simulink model "W2G_ss_lupa"  (R2021b)
settings: Solver=ode4  StartTime=0  StopTime=10  FixedStep=0.1  MaxStep=0.1  RelTol=1e-3  EnableMultiTasking=on
undefined symbols (not defined in the file): absPower, body, constraint, elecPower, ess, force, fricForce, geometry, gsc, hydroData, Ia, Ib, Ic, mooring, Pgen, Pgrid, pto, ptoSim, Qgrid_lim, simu, Va, Vb, Vc, Vdc, vel, waves, wsc, X, Y, Z
libraries: sm_lib x8, WECSim_Lib_Body_Elements x2, nesl_utility x2, simulink x1, WECSim_Lib_Moorings x1, WECSim_Lib_PTOs x1, WECSim_Lib_Constraints x1
settings Model: Creator=mlawson  LastModifiedBy=alexb
settings SolverCC: ZeroCrossControl=DisableAll  AlgebraicLoopSolver=LineSearch  AutoInsertRateTranBlk=on
settings DataIOCC: SaveFormat=Array  SaveOutput=off  SaveTime=off  ReturnWorkspaceOutputs=off
settings OptimizationCC: LifeSpan=inf  SimCompilerOptimization=on
settings DebuggingCC: UnderspecifiedInitializationDetection=Classic  MergeDetectMultiDrivingBlocksExec=none  SolverPrmCheckMsg=warning  AllowSymbolicDim=off  StateNameClashWarn=warning  SFUnexpectedBacktrackingDiag=warning  SFNoUnconditionalDefaultTransitionDiag=warning  SFMachineParentedDataDiag=warning  ArithmeticOperatorsInVariantConditions=warning
settings HardwareCC: ProdBitPerPointer=32  ProdBitPerSizeT=32  ProdBitPerPtrDiffT=32  ProdLargestAtomicFloat=None  ProdIntDivRoundTo=Undefined  ProdEndianess=Unspecified  ProdWordSize=32  ProdHWDeviceType=32-bit Generic
settings ModelReferenceCC: PropagateSignalLabelsOutOfModel=off
settings SFSimCC: SimUseLocalCustomCode=off  CustomCodeUndefinedFunction=UseInterfaceOnly
settings RTWCC: RTWUseLocalCustomCode=off
settings CodeAppCC: StateflowObjectComments=on
settings GRTTargetCC: TargetLangStandard=C89/C90 (ANSI)
settings ConfigComp: CovMetricSettings=dw  CovSaveCumulativeToWorkspaceVar=on  CovSaveSingleToWorkspaceVar=on  CovExternalEMLEnable=off  CovSFcnEnable=off
settings SimscapeCC: SimscapeNormalizeSystem=off
settings ConfigurationSet: Description=SimMechanics 2G
settings ExplorerConfigSet: SimMechanicsOpenEditorOnUpdate=off  InternalSimMechanicsExplorerSettings="<ExplorerConfiguration><canonicalview>default</canonicalview><TilePanel><TileInfo><Tiles Columns=\"1\" Count=\"1\" Rows=\"1\"><Column Left=\"2\" Weight=\"1\"/><Column Left=\"1335\"/><Row Top=\"2\" Weight=\"1\"/><Row Top=\"911\"/><Tile Height=\"1\" Width=\"1\" X=\"0\" Y=\"0\"/></Tiles></TileInfo><SceneInfo><SceneViewer><BGColor><R>0.60000002384185791</R><G>0.60000002384185791</G><B>0.60000002384185791</B></BGColor><Camera><Position><X>365.37645888990272</X><Y>-369.82486814446582</Y><Z>359.64809521743916</Z></Position><Center><X>-6.7351450971904585</X><Y>2.2867358426280204</Y><Z>-12.463508769654169</Z></Center><Up><X>-0.40824829046386307</X><Y>0.40824829046386307</Y><Z>0.81649658092772615</Z></Up><Left>-57.820127362122818</Left><Right>57.820127362122818</Right><Bottom>-38.308817187253304</Bottom><Top>38.308817187253304</Top></Camera></SceneViewer></SceneInfo></TilePanel></ExplorerConfiguration>"

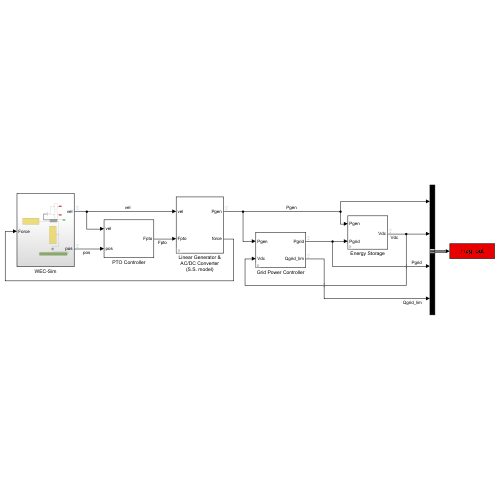
[thumbnail: Simulink's stored preview of the top-level diagram]
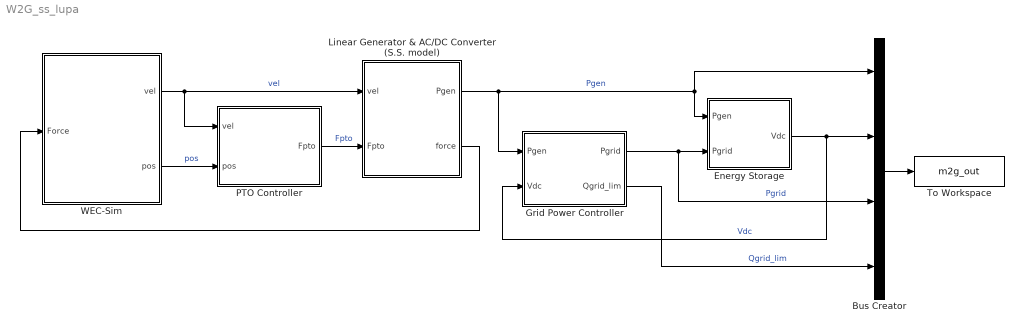
== system W2G_ss_lupa ==
  Bus Creator : BusCreator  Inputs=Pgen,Vdc,Pgrid,Qgrid_lim
  Energy Storage : Subsystem  mask{Vdc_0=ess.Vdc_0, C=ess.C}
      mask prompts: Vdc_0 "Initial Voltage"; C "Capacitance (C):"
      mask DialogControl DescTextVar_copy Prompt: Uses classical SC model.
      mask DialogControl ParamGroupVar Prompt: SC Bank Parameters
  Grid Power Controller : Subsystem  mask{Tavg=gsc.Tavg, Vmag=gsc.Vmag, Ilim=gsc.Ilim, Prated=gsc.Prated, Vdc_nom=ess.Vdc_0, Vdc_del=ess.Vdc_del, kp_v=gsc.kp, ki_v=gsc.ki}
      mask prompts: Tavg "Averaging Time Constant (s):"; Vmag "Grid voltage magnitude (V):"; Ilim "GSC current limit (A):"; Prated "GSC rated power (W):"; Vdc_nom "DC link nominal voltage (V):"; Vdc_del "DC link voltage deviation maximum (V):"; kp_v "Voltage regulator proportional gain:"; ki_v "Voltage regulator integral gain:"
  Linear Generator & AC/DC Converter (S.S. model) : Subsystem  mask{ptoSim=ptoSim.directLinearGenerator(1)}
      mask prompts: ptoSim "Machine Name"
  PTO Controller : Subsystem
  To Workspace : ToWorkspace  VariableName=m2g_out  SaveFormat=Timeseries  SampleTime=-1
  WEC-Sim : Subsystem
  wires:
  WEC-Sim/1(vel) -> PTO Controller/1(vel), Linear Generator & AC/DC Converter (S.S. model)/1(vel)  "vel"
  Linear Generator & AC/DC Converter (S.S. model)/2(force) -> WEC-Sim/1(Force)
  Linear Generator & AC/DC Converter (S.S. model)/1(Pgen) -> Grid Power Controller/1(Pgen), Bus Creator/1, Energy Storage/1(Pgen)  "Pgen"
  Grid Power Controller/1(Pgrid) -> Bus Creator/3, Energy Storage/2(Pgrid)  "Pgrid"
  Grid Power Controller/2(Qgrid_lim) -> Bus Creator/4  "Qgrid_lim"
  Energy Storage/1(Vdc) -> Grid Power Controller/2(Vdc), Bus Creator/2  "Vdc"
  WEC-Sim/2(pos) -> PTO Controller/2(pos)  "pos"
  PTO Controller/1(Fpto) -> Linear Generator & AC/DC Converter (S.S. model)/2(Fpto)  "Fpto"
  Bus Creator/1 -> To Workspace/1

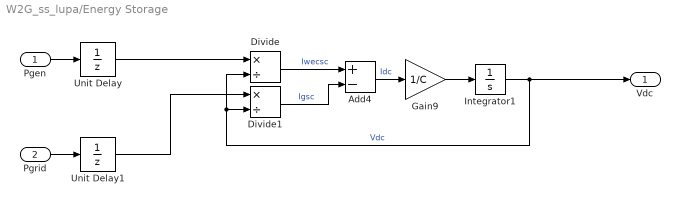
== system W2G_ss_lupa/Energy Storage ==
  Pgen : Inport
  Pgrid : Inport  Port=2
  Add4 : Sum  Inputs=+-
  Divide : Product  Inputs=*/
  Divide1 : Product  Inputs=*/
  Gain9 : Gain  Gain=1/C
  Integrator1 : Integrator  InitialCondition=Vdc_0
  Unit Delay : UnitDelay  SampleTime=-1  HasFrameUpgradeWarning=on
  Unit Delay1 : UnitDelay  SampleTime=-1  HasFrameUpgradeWarning=on
  Vdc : Outport
  wires:
  Pgen/1 -> Unit Delay/1
  Add4/1 -> Gain9/1  "Idc"
  Divide/1 -> Add4/1  "Iwecsc"
  Gain9/1 -> Integrator1/1
  Integrator1/1 -> Vdc/1, Divide1/2, Divide/2  "Vdc"
  Divide1/1 -> Add4/2  "Igsc"
  Pgrid/1 -> Unit Delay1/1
  Unit Delay/1 -> Divide/1
  Unit Delay1/1 -> Divide1/1

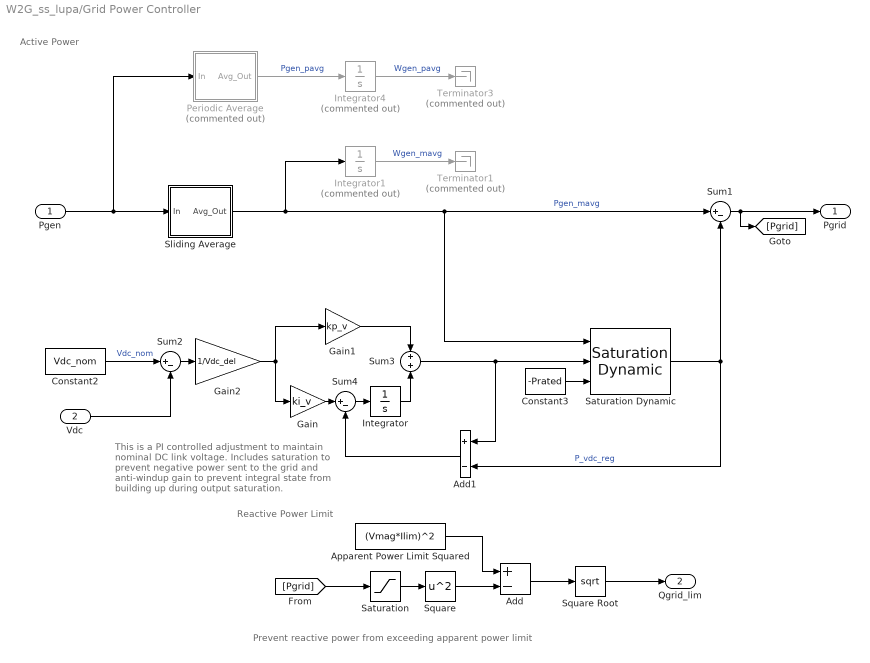
== system W2G_ss_lupa/Grid Power Controller ==
  note: This is a PI controlled adjustment to maintain nominal DC link voltage. Includes saturation to prevent negative power sent to the grid and anti-windup gain to prevent integral state from building up during output saturation.
  note: Reactive Power Limit
  note: Active Power
  note: Prevent reactive power from exceeding apparent power limit
  Pgen : Inport
  Vdc : Inport  Port=2
  Add : Sum  Inputs=+-
  Add1 : Sum  Inputs=+-
  Apparent Power Limit Squared : Constant  Value=(Vmag*Ilim)^2
  Constant2 : Constant  Value=Vdc_nom
  Constant3 : Constant  Value=-Prated
  Gain : Gain  Gain=ki_v
  Gain1 : Gain  Gain=kp_v
  Gain2 : Gain  Gain=1/Vdc_del
  Integrator : Integrator
  Integrator1 : Integrator  Commented=on
  Integrator4 : Integrator  Commented=on
  Periodic Average : Subsystem  Commented=on  mask{Tsample=Tavg}
      mask prompts: Tsample "Sampling Period (s):"
  Saturation : Saturate  UpperLimit=Vmag*Ilim  LowerLimit=-Vmag*Ilim
  Saturation Dynamic : simulink/Discontinuities/Saturation Dynamic  OutMin=[]  OutMax=[]  OutDataTypeStr=Inherit: Same as second input  OutDataType=fixdt(1, 16)  OutScaling=2^-10  DoSatur=off
  Sliding Average : Subsystem  mask{Tsample=Tavg, dt=simu.dt}
      mask prompts: Tsample "Sampling Period (s):"; dt "Simulation Time Step (s):"
  Square : Math  Operator=square  SaturateOnIntegerOverflow=on
  Square Root : Sqrt  SaturateOnIntegerOverflow=on
  Sum1 : Sum  Inputs=|+-
  Sum2 : Sum  Inputs=|+-
  Sum3 : Sum
  Sum4 : Sum  Inputs=|+-
  Terminator1 : Terminator  Commented=on
  Terminator3 : Terminator  Commented=on
  Pgrid : Outport
  Qgrid_lim : Outport  Port=2
  wires:
  Pgen/1 -> Periodic Average/1(In), Sliding Average/1(In)
  Integrator4/1 -> Terminator3/1  "Wgen_pavg"
  Integrator1/1 -> Terminator1/1  "Wgen_mavg"
  Sliding Average/1(Avg_Out) -> Saturation Dynamic/1, Sum1/1, Integrator1/1  "Pgen_mavg"
  Periodic Average/1(Avg_Out) -> Integrator4/1  "Pgen_pavg"
  Add/1 -> Square Root/1
  Square/1 -> Add/2
  Saturation/1 -> Square/1
  Square Root/1 -> Qgrid_lim/1
  Apparent Power Limit Squared/1 -> Add/1
  Sum1/1 -> [Pgrid], Pgrid/1
  [Pgrid] -> Saturation/1
  Constant2/1 -> Sum2/1  "Vdc_nom"
  Constant3/1 -> Saturation Dynamic/3
  Sum3/1 -> Add1/1, Saturation Dynamic/2
  Gain1/1 -> Sum3/1
  Integrator/1 -> Sum3/2
  Saturation Dynamic/1 -> Add1/2, Sum1/2  "P_vdc_reg"
  Vdc/1 -> Sum2/2
  Sum2/1 -> Gain2/1
  Gain2/1 -> Gain1/1, Gain/1
  Gain/1 -> Sum4/1
  Sum4/1 -> Integrator/1
  Add1/1 -> Sum4/2

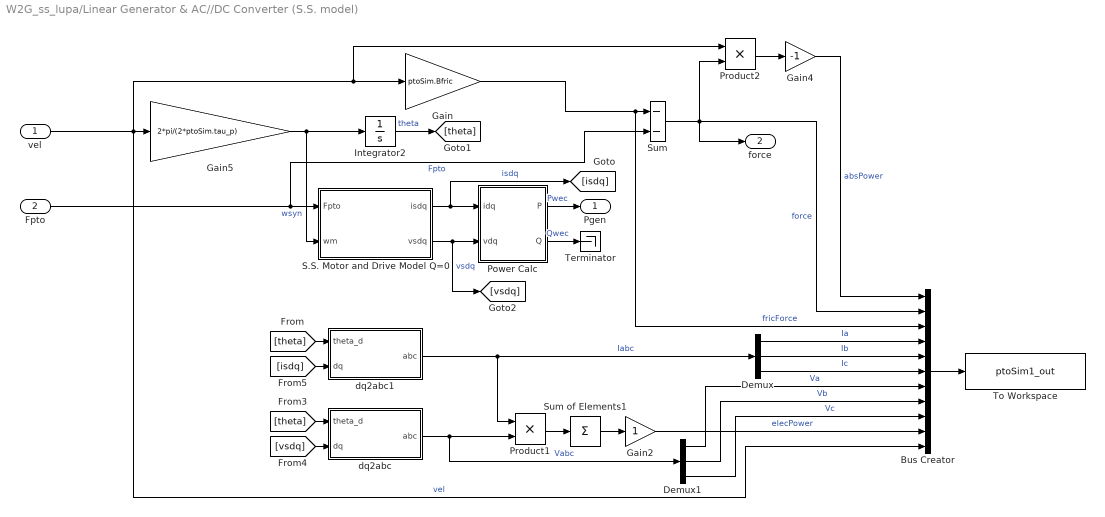
== system W2G_ss_lupa/Linear Generator & AC//DC Converter (S.S. model) ==
  vel : Inport
  Fpto : Inport  Port=2
  Bus Creator : BusCreator  Inputs=absPower,force,fricForce,Ia,Ib,Ic,Va,Vb,Vc,elecPower,vel
  Demux : Demux  Outputs=3
  Demux1 : Demux  Outputs=3
  Gain : Gain  Gain=ptoSim.Bfric
  Gain2 : Gain
  Gain4 : Gain  Gain=-1
  Gain5 : Gain  Gain=2*pi/(2*ptoSim.tau_p)
  Integrator2 : Integrator  InitialCondition=ptoSim.theta_d_0
  Power Calc : Subsystem
  Product1 : Product
  Product2 : Product
  S.S. Motor and Drive Model Q=0 : Subsystem
  Sum : Sum  Inputs=--
  Sum of Elements1 : Sum  Inputs=+
  Terminator : Terminator
  To Workspace : ToWorkspace  VariableName=ptoSim1_out  SaveFormat=Structure With Time  SampleTime=simu.dtOut
  dq2abc : Subsystem
  dq2abc1 : Subsystem
  Pgen : Outport
  force : Outport  Port=2
  wires:
  Gain/1 -> Sum/1, Bus Creator/3  "fricForce"
  S.S. Motor and Drive Model Q=0/2(vsdq) -> [vsdq], Power Calc/2(vdq)  "vsdq"
  Sum/1 -> Product2/2, force/1, Bus Creator/2  "force"
  Sum of Elements1/1 -> Gain2/1
  Integrator2/1 -> [theta]  "theta"
  vel/1 -> Gain/1, Product2/1, Bus Creator/11, Gain5/1  "vel"
  Gain2/1 -> Bus Creator/10  "elecPower"
  Product1/1 -> Sum of Elements1/1
  dq2abc/1(abc) -> Demux1/1, Product1/2  "Vabc"
  Demux1/3 -> Bus Creator/9  "Vc"
  Demux1/2 -> Bus Creator/8  "Vb"
  Demux/3 -> Bus Creator/6  "Ic"
  Gain5/1 -> Integrator2/1, S.S. Motor and Drive Model Q=0/2(wm)  "wsyn"
  Demux1/1 -> Bus Creator/7  "Va"
  Demux/1 -> Bus Creator/4  "Ia"
  S.S. Motor and Drive Model Q=0/1(isdq) -> Power Calc/1(idq), [isdq]  "isdq"
  Bus Creator/1 -> To Workspace/1
  Demux/2 -> Bus Creator/5  "Ib"
  dq2abc1/1(abc) -> Product1/1, Demux/1  "Iabc"
  Gain4/1 -> Bus Creator/1  "absPower"
  Product2/1 -> Gain4/1
  Power Calc/2(Q) -> Terminator/1  "Qwec"
  Power Calc/1(P) -> Pgen/1  "Pwec"
  [theta] -> dq2abc1/1(theta_d)
  [theta] -> dq2abc/1(theta_d)
  [vsdq] -> dq2abc/2(dq)
  [isdq] -> dq2abc1/2(dq)
  Fpto/1 -> S.S. Motor and Drive Model Q=0/1(Fpto), Sum/2  "Fpto"

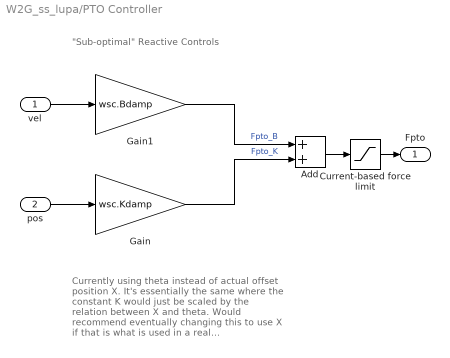
== system W2G_ss_lupa/PTO Controller ==
  note: "Sub-optimal" Reactive Controls
  note: Currently using theta instead of actual offset position X. It's essentially the same where the constant K would just be scaled by the relation between X and theta. Would recommend eventually changing this to use X if that is what is used in a real implementation.
  vel : Inport
  pos : Inport  Port=2
  Add : Sum
  Current-based force limit : Saturate  UpperLimit=wsc.Fpto_lim  LowerLimit=-wsc.Fpto_lim
  Gain : Gain  Gain=wsc.Kdamp
  Gain1 : Gain  Gain=wsc.Bdamp
  Fpto : Outport
  wires:
  Gain1/1 -> Add/1  "Fpto_B"
  Gain/1 -> Add/2  "Fpto_K"
  vel/1 -> Gain1/1
  pos/1 -> Gain/1
  Add/1 -> Current-based force limit/1
  Current-based force limit/1 -> Fpto/1

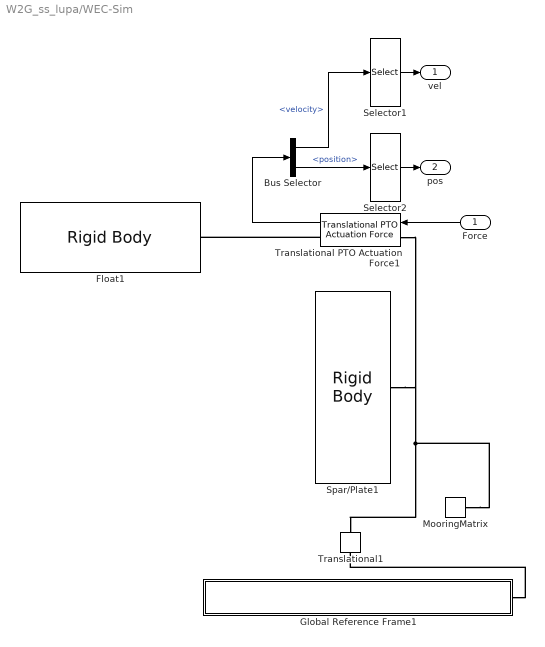
== system W2G_ss_lupa/WEC-Sim ==
  Force : Inport
  Bus Selector : BusSelector  OutputSignals=velocity,position
  Float1 : WECSim_Lib_Body_Elements/Rigid Body  body=body(1)  h5File=hydroData/*.h5  geometryFile=geometry/*.stl  mass=0  inertia=0 0 0  nonHydro=0  nonlinearHydro=0  centerGravity=0 0 0  centerBuoyancy=0 0 0  dof=6  volume=0  displacement=0 0 0  axis=0 1 0  angle=0  option=0  cd=0 0 0  ca=0 0 0  area=0 0 0  VME=0  rgME=0 0 0  z=0 0 1
      settings: SourceProductName=WEC-Sim
  Global Reference Frame1 : Subsystem  AncestorBlock=WECSim_Lib_Frames/Global Reference Frame  StopFcn=%run('stopWecSim')  mask(Frames){waves=waves, simu=simu, InputMethod=Input File, InputFile=wecSimInputFile.m, mode=normal, explorer=off, solver=ode4, startTime=0, rampTime=100, endTime=400, dt=0.1, cicEndTime=60, stateSpace=0, WaveClass=regular, height=2.5, period=8, elevationFile=NOT DEFINED, spectrumFile=NOT DEFINED, direction=0, spread=1, spectrumType=NOT DEFINED, phaseSeed=0, option=EqualEnergy}
      mask prompts: waves "Wave Class Name"; simu "Simulation Class Name"; InputMethod "Parameter Input Method"; mode "Simulation Mode:"; explorer "SimMechanics Explorer:"; solver "SimSolver:"; startTime "Start Time [s]:"; rampTime "Ramp Time [s]:"; endTime "End Time [s]:"; dt "Step Size [s]:"; cicEndTime "CI Time [s]:"; stateSpace "Turn on State Space"; WaveClass "Select Wave Class:"; height "Wave Height [m]:"; period "Wave Period [s]:"; direction "Wave Direction [deg]:"; spread "Wave Spread [0-1]:"; spectrumType "Wave Spectrum Type:"; phaseSeed "Phase Seed:"; option "Frequency Discretization:"
      mask help:
      | This block contains Global References, including solver configurations, free surface and seabed description, and simulation time.
      | It uses the following fields from the Simulation and Wave classes:
      |
      | Simulation Class:
      |     .endTime
      |     .dt
      |     .domainSize
      |
      | Wave Class:
      |     .waterDepth
      mask Help:
      | This block contains Global References, including solver configurations, free surface and seabed description, and simulation time.
      | It uses the following fields from the Simulation and Wave classes:
      | 
      | Simulation Class:
      |     .endTime
      |     .dt
      |     .domainSize
      | 
      | Wave Class:
      |     .waterDepth
      mask TypeOptions InputMethod: Input File | Custom Parameters
      mask Callback InputMethod: inputOrCustomCallback(gcbh)
      mask TypeOptions mode: normal | accelerator | rapid-accelerator
      mask TypeOptions explorer: on | off
      mask TypeOptions solver: ode4 | ode45
      mask TypeOptions stateSpace: 0 | 1
      mask TypeOptions WaveClass: noWaveCIC | regular | regularCIC | irregular | spectrumImport | etaImport
      mask Callback WaveClass: waveClassCallback(gcbh)
      mask TypeOptions spectrumType: PM | JS | NOT DEFINED
      mask TypeOptions option: EqualEnergy | Traditional
      mask DialogControl InputFileGroup Prompt: Input File
      mask DialogControl InFileButton Prompt: Select File
      mask DialogControl InFileButton Callback: inFileButtonCallback(gcbh)
      mask DialogControl CustomParameterGroup Prompt: Custom Parameters
      mask DialogControl LoadParam Prompt: Load parameters from Input File
      mask DialogControl LoadParam Callback: loadInputFileCallback(gcbh)
      mask DialogControl SimData Prompt: Simulation Data
      mask DialogControl WaveInfo Prompt: Wave Information
      mask DialogControl ETAbutton Prompt: Select etaData.mat file
      mask DialogControl ETAbutton Callback: etaButtonCallback(gcbh)
      mask DialogControl SpecButton Prompt: Select spectrumData.mat file
      mask DialogControl SpecButton Callback: spectrumButtonCallback(gcbh)
      mask Display: fprintf('Active Method: \n%s',get_param(gcbh,'InputMethod'))
  MooringMatrix : WECSim_Lib_Moorings/MooringMatrix  mooring=mooring(1)  loc=0 0 0  preTension=[0 0 0 0 0 0]  stiffness={ '0', '0', '0', '0', '0', '0'; '0', '0', '0', '0', '0', '0'; '0', '0', '0', '0', '0', '0'; '0', '0', '0', '0', '0', '0'; '0', '0', '0', '0', '0', '0'; '0', '0', '0', '0', '0', '0' }  damping={ '0', '0', '0', '0', '0', '0'; '0', '0', '0', '0', '0', '0'; '0', '0', '0', '0', '0', '0'; '0', '0', '0', '0', '0', '0'; '0', '0', '0', '0', '0', '0'; '0', '0', '0', '0', '0', '0' }
      settings: AttributesFormatString=%<mooring>
  Selector1 : Selector  InputPortWidth=6  IndexOptions=Index vector (dialog)  Indices=3  OutputSizes=1
  Selector2 : Selector  InputPortWidth=6  IndexOptions=Index vector (dialog)  Indices=3  OutputSizes=1
  Spar/Plate1 : WECSim_Lib_Body_Elements/Rigid Body  body=body(2)  h5File=hydroData/*.h5  geometryFile=geometry/*.stl  mass=0  inertia=0 0 0  nonHydro=0  nonlinearHydro=0  centerGravity=0 0 0  centerBuoyancy=0 0 0  dof=6  volume=0  displacement=0 0 0  axis=0 1 0  angle=0  option=0  cd=0 0 0  ca=0 0 0  area=0 0 0  VME=0  rgME=0 0 0  z=0 0 1
      settings: SourceProductName=WEC-Sim
  Translational PTO Actuation Force1 : WECSim_Lib_PTOs/Translational PTO Actuation Force  pto=pto(1)  loc="0  0  0"  stiffness=0  damping=0  equilibriumPosition=0  pretension=0  displacement=0 0 0  y=0 1 0  z=0 0 1  upperLimitSpecify=off  upperLimitBound=0  upperLimitTransitionRegionWidth=0  upperLimitStiffness=0  upperLimitDamping=0  lowerLimitSpecify=off  lowerLimitBound=0  lowerLimitTransitionRegionWidth=0  lowerLimitStiffness=0  lowerLimitDamping=0
      settings: AttributesFormatString=%<pto>  SourceProductName=WEC-Sim
  Translational1 : WECSim_Lib_Constraints/Translational  constraint=constraint(1)  loc="0  0  0"  displacement=0 0 0  y=0 1 0  z=0 0 1  upperLimitSpecify=off  upperLimitBound=0  upperLimitTransitionRegionWidth=0  upperLimitStiffness=0  upperLimitDamping=0  lowerLimitSpecify=off  lowerLimitBound=0  lowerLimitTransitionRegionWidth=0  lowerLimitStiffness=0  lowerLimitDamping=0
      settings: AttributesFormatString=%<constraint>  SourceProductName=WEC-Sim
  vel : Outport
  pos : Outport  Port=2
  wires:
  Force/1 -> Translational PTO Actuation Force1/1
  Selector1/1 -> vel/1
  Bus Selector/1 -> Selector1/1  "<velocity>"
  Translational PTO Actuation Force1/1 -> Bus Selector/1
  Bus Selector/2 -> Selector2/1  "<position>"
  Selector2/1 -> pos/1
  connections:
  Spar/Plate1/RConn1 -- Translational PTO Actuation Force1/LConn1 -- MooringMatrix/LConn1 -- Translational1/RConn1
  Translational PTO Actuation Force1/RConn1 -- Float1/RConn1
  Global Reference Frame1/RConn1 -- Translational1/LConn1

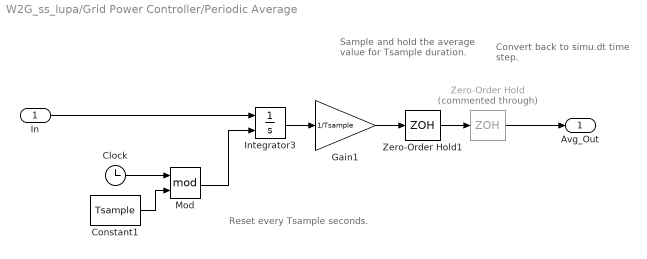
== system W2G_ss_lupa/Grid Power Controller/Periodic Average ==
  note: Reset every Tsample seconds.
  note: Convert back to simu.dt time step.
  note: Sample and hold the average value for Tsample duration.
  In : Inport
  Clock : Clock
  Constant1 : Constant  Value=Tsample
  Gain1 : Gain  Gain=1/Tsample
  Integrator3 : Integrator  ExternalReset=rising
  Mod : Math  Operator=mod  OutputSignalType=real  SaturateOnIntegerOverflow=on
  Zero-Order Hold : ZeroOrderHold  Commented=through  SampleTime=simu.dt
  Zero-Order Hold1 : ZeroOrderHold  SampleTime=Tsample
  Avg_Out : Outport
  wires:
  Zero-Order Hold/1 -> Avg_Out/1
  Mod/1 -> Integrator3/2
  Zero-Order Hold1/1 -> Zero-Order Hold/1
  Clock/1 -> Mod/1
  Gain1/1 -> Zero-Order Hold1/1
  Integrator3/1 -> Gain1/1
  In/1 -> Integrator3/1
  Constant1/1 -> Mod/2

== system W2G_ss_lupa/Grid Power Controller/Sliding Average ==
  In : Inport
  Discrete FIR Filter : DiscreteFir  Coefficients=ones(1,round(Tsample/dt))/round(Tsample/dt)  SampleTime=dt
  Avg_Out : Outport
  wires:
  In/1 -> Discrete FIR Filter/1
  Discrete FIR Filter/1 -> Avg_Out/1

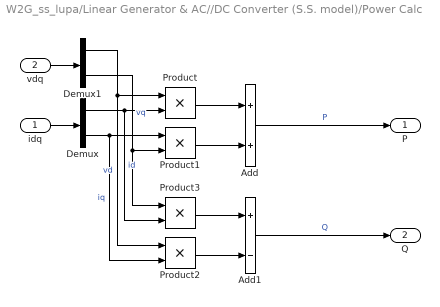
== system W2G_ss_lupa/Linear Generator & AC//DC Converter (S.S. model)/Power Calc ==
  idq : Inport
  vdq : Inport  Port=2
  Add : Sum
  Add1 : Sum  Inputs=+-
  Demux : Demux  Outputs=2
  Demux1 : Demux  Outputs=2
  Product{,1..3} (4 alike) : Product
  P : Outport
  Q : Outport  Port=2
  wires:
  Demux/1 -> Product3/2, Product/2  "id"
  Product1/1 -> Add/2
  Add1/1 -> Q/1  "Q"
  Demux1/2 -> Product1/2, Product3/1  "vq"
  Demux1/1 -> Product/1, Product2/1  "vd"
  Demux/2 -> Product2/2, Product1/1  "iq"
  Product3/1 -> Add1/1
  Product2/1 -> Add1/2
  Product/1 -> Add/1
  Add/1 -> P/1  "P"
  idq/1 -> Demux/1
  vdq/1 -> Demux1/1

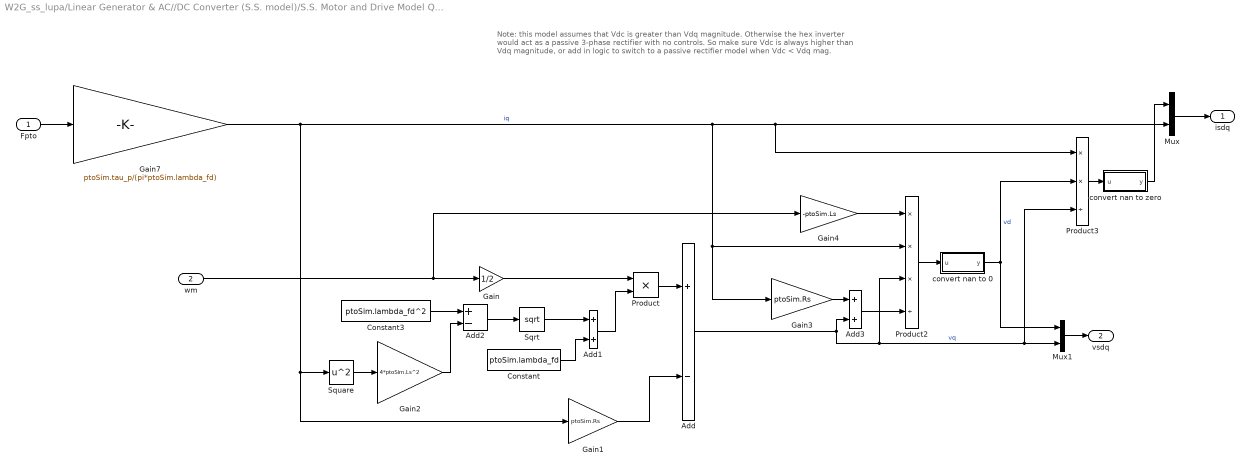
== system W2G_ss_lupa/Linear Generator & AC//DC Converter (S.S. model)/S.S. Motor and Drive Model Q=0 ==
  note: Note: this model assumes that Vdc is greater than Vdq magnitude. Otherwise the hex inverter would act as a passive 3-phase rectifier with no controls. So make sure Vdc is always higher than Vdq magnitude, or add in logic to switch to a passive rectifier model when Vdc < Vdq mag.
  Fpto : Inport
  wm : Inport  Port=2
  Add : Sum  Inputs=+-
  Add1 : Sum
  Add2 : Sum  Inputs=+-
  Add3 : Sum
  Constant : Constant  Value=ptoSim.lambda_fd
  Constant3 : Constant  Value=ptoSim.lambda_fd^2
  Gain : Gain  Gain=1/2
  Gain1 : Gain  Gain=ptoSim.Rs
  Gain2 : Gain  Gain=4*ptoSim.Ls^2
  Gain3 : Gain  Gain=ptoSim.Rs
  Gain4 : Gain  Gain=-ptoSim.Ls
  Gain7 : Gain  Gain=ptoSim.tau_p/(pi*ptoSim.lambda_fd)
  Mux : Mux  Inputs=2
  Mux1 : Mux  Inputs=2
  Product : Product
  Product2 : Product  Inputs=***/
  Product3 : Product  Inputs=**/
  Sqrt : Sqrt  SaturateOnIntegerOverflow=on
  Square : Math  Operator=square  SaturateOnIntegerOverflow=on
  convert nan to 0 : MATLAB Function  TreatAsAtomicUnit=on
  convert nan to zero : MATLAB Function  TreatAsAtomicUnit=on
  isdq : Outport
  vsdq : Outport  Port=2
  wires:
  Fpto/1 -> Gain7/1
  Mux/1 -> isdq/1
  Mux1/1 -> vsdq/1
  Gain7/1 -> Product2/2, Gain3/1, Product3/1, Mux/2, Gain1/1, Square/1  "iq"
  Constant/1 -> Add1/2
  convert nan to 0/1(y) -> Product3/2, Mux1/1  "vd"
  Add/1 -> Product2/3, Product3/3, Mux1/2, Add3/2  "vq"
  convert nan to zero/1(y) -> Mux/1
  Gain1/1 -> Add/2
  Product/1 -> Add/1
  Gain/1 -> Product/1
  Add1/1 -> Product/2
  Sqrt/1 -> Add1/1
  Add2/1 -> Sqrt/1
  Constant3/1 -> Add2/1
  Gain2/1 -> Add2/2
  Product2/1 -> convert nan to 0/1(u)
  Add3/1 -> Product2/4
  Gain3/1 -> Add3/1
  Gain4/1 -> Product2/1
  Product3/1 -> convert nan to zero/1(u)
  Square/1 -> Gain2/1
  wm/1 -> Gain4/1, Gain/1

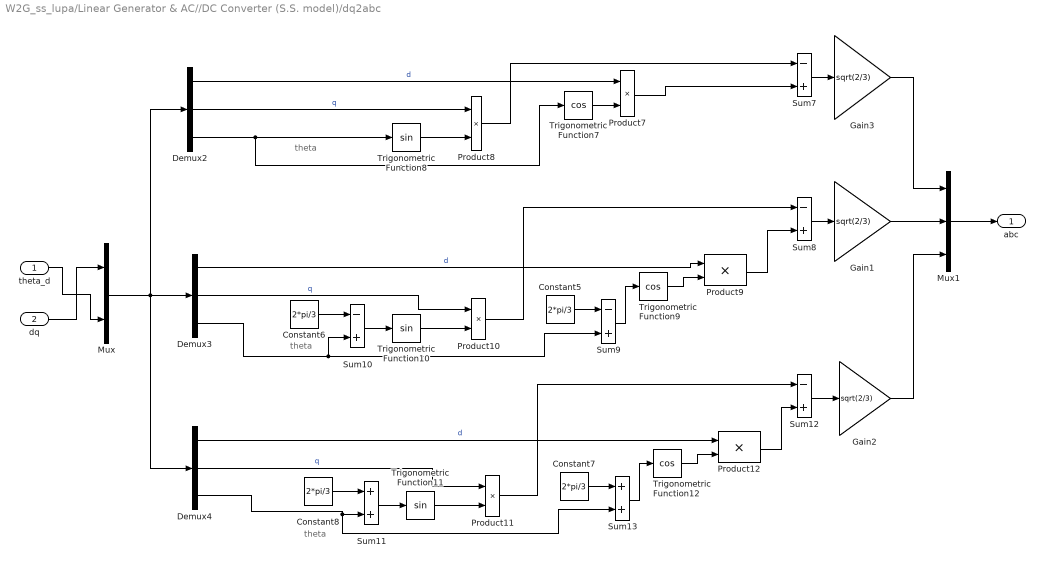
== system W2G_ss_lupa/Linear Generator & AC//DC Converter (S.S. model)/dq2abc ==
  note: theta
  note: theta
  note: theta
  theta_d : Inport
  dq : Inport  Port=2
  Constant{5..8} (4 alike) : Constant  Value=2*pi/3
  Demux2 : Demux  Outputs=3
      settings: DisplayOption=none
  Demux3 : Demux  Outputs=3
      settings: DisplayOption=none
  Demux4 : Demux  Outputs=3
      settings: DisplayOption=none
  Gain1 : Gain  Gain=sqrt(2/3)  SaturateOnIntegerOverflow=on  OutDataTypeStr=Inherit: Same as input  ParamDataTypeStr=Inherit: Same as input
  Gain2 : Gain  Gain=sqrt(2/3)  SaturateOnIntegerOverflow=on  OutDataTypeStr=Inherit: Same as input  ParamDataTypeStr=Inherit: Same as input
  Gain3 : Gain  Gain=sqrt(2/3)  SaturateOnIntegerOverflow=on  OutDataTypeStr=Inherit: Same as input  ParamDataTypeStr=Inherit: Same as input
  Mux : Mux  Inputs=2
  Mux1 : Mux  Inputs=3
  Product{7..12} (6 alike) : Product  InputSameDT=on  SaturateOnIntegerOverflow=on  OutDataTypeStr=Inherit: Same as first input
  Sum{7..10,12} (5 alike) : Sum  Inputs=-+  InputSameDT=on  SaturateOnIntegerOverflow=on  OutDataTypeStr=Inherit: Same as first input
  Sum11 : Sum  InputSameDT=on  SaturateOnIntegerOverflow=on  OutDataTypeStr=Inherit: Same as first input
  Sum13 : Sum  InputSameDT=on  SaturateOnIntegerOverflow=on  OutDataTypeStr=Inherit: Same as first input
  Trigonometric Function10 : Trigonometry
  Trigonometric Function11 : Trigonometry
  Trigonometric Function12 : Trigonometry  Operator=cos
  Trigonometric Function7 : Trigonometry  Operator=cos
  Trigonometric Function8 : Trigonometry
  Trigonometric Function9 : Trigonometry  Operator=cos
  abc : Outport
  wires:
  Constant8/1 -> Sum11/1
  Product7/1 -> Sum7/2
  Gain1/1 -> Mux1/2
  Product9/1 -> Sum8/2
  Sum7/1 -> Gain3/1
  Demux4/2 -> Product11/1  "q"
  Product10/1 -> Sum8/1
  Product11/1 -> Sum12/1
  Sum13/1 -> Trigonometric Function12/1
  Demux2/3 -> Trigonometric Function7/1, Trigonometric Function8/1
  Product12/1 -> Sum12/2
  Constant6/1 -> Sum10/1
  Product8/1 -> Sum7/1
  Mux1/1 -> abc/1
  Demux3/3 -> Sum9/2, Sum10/2
  Demux3/2 -> Product10/1  "q"
  Demux2/2 -> Product8/1  "q"
  dq/1 -> Mux/1
  Trigonometric Function7/1 -> Product7/2
  Constant5/1 -> Sum9/1
  Trigonometric Function12/1 -> Product12/2
  Trigonometric Function10/1 -> Product10/2
  Demux4/1 -> Product12/1  "d"
  Gain2/1 -> Mux1/3
  Demux4/3 -> Sum11/2, Sum13/2
  Demux2/1 -> Product7/1  "d"
  Sum10/1 -> Trigonometric Function10/1
  Gain3/1 -> Mux1/1
  Mux/1 -> Demux3/1, Demux2/1, Demux4/1
  Sum12/1 -> Gain2/1
  theta_d/1 -> Mux/2
  Sum11/1 -> Trigonometric Function11/1
  Trigonometric Function9/1 -> Product9/2
  Sum8/1 -> Gain1/1
  Sum9/1 -> Trigonometric Function9/1
  Demux3/1 -> Product9/1  "d"
  Trigonometric Function8/1 -> Product8/2
  Trigonometric Function11/1 -> Product11/2
  Constant7/1 -> Sum13/1

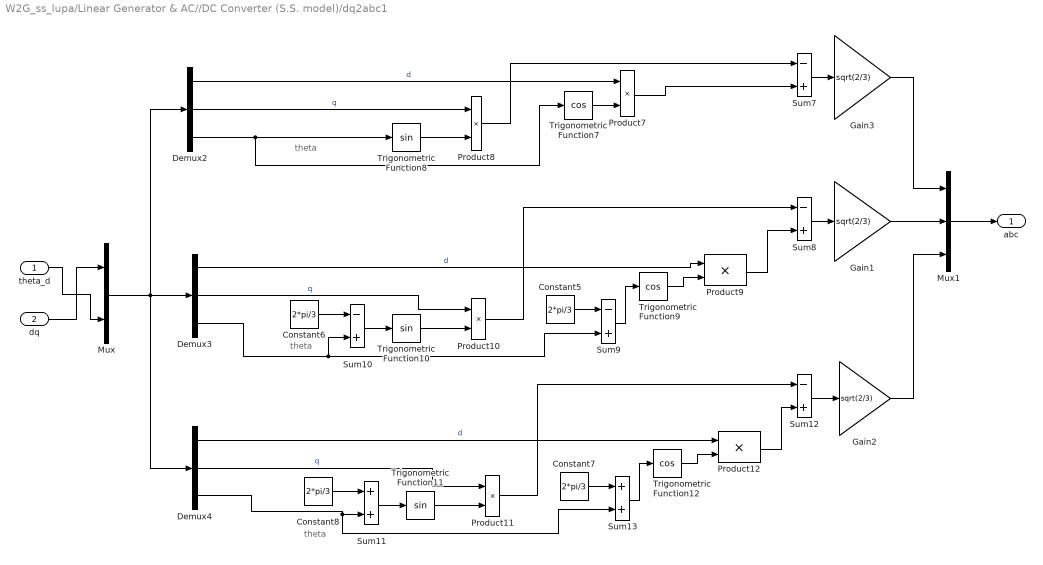
== system W2G_ss_lupa/Linear Generator & AC//DC Converter (S.S. model)/dq2abc1 ==
  note: theta
  note: theta
  note: theta
  theta_d : Inport
  dq : Inport  Port=2
  Constant{5..8} (4 alike) : Constant  Value=2*pi/3
  Demux2 : Demux  Outputs=3
      settings: DisplayOption=none
  Demux3 : Demux  Outputs=3
      settings: DisplayOption=none
  Demux4 : Demux  Outputs=3
      settings: DisplayOption=none
  Gain1 : Gain  Gain=sqrt(2/3)  SaturateOnIntegerOverflow=on  OutDataTypeStr=Inherit: Same as input  ParamDataTypeStr=Inherit: Same as input
  Gain2 : Gain  Gain=sqrt(2/3)  SaturateOnIntegerOverflow=on  OutDataTypeStr=Inherit: Same as input  ParamDataTypeStr=Inherit: Same as input
  Gain3 : Gain  Gain=sqrt(2/3)  SaturateOnIntegerOverflow=on  OutDataTypeStr=Inherit: Same as input  ParamDataTypeStr=Inherit: Same as input
  Mux : Mux  Inputs=2
  Mux1 : Mux  Inputs=3
  Product{7..12} (6 alike) : Product  InputSameDT=on  SaturateOnIntegerOverflow=on  OutDataTypeStr=Inherit: Same as first input
  Sum{7..10,12} (5 alike) : Sum  Inputs=-+  InputSameDT=on  SaturateOnIntegerOverflow=on  OutDataTypeStr=Inherit: Same as first input
  Sum11 : Sum  InputSameDT=on  SaturateOnIntegerOverflow=on  OutDataTypeStr=Inherit: Same as first input
  Sum13 : Sum  InputSameDT=on  SaturateOnIntegerOverflow=on  OutDataTypeStr=Inherit: Same as first input
  Trigonometric Function10 : Trigonometry
  Trigonometric Function11 : Trigonometry
  Trigonometric Function12 : Trigonometry  Operator=cos
  Trigonometric Function7 : Trigonometry  Operator=cos
  Trigonometric Function8 : Trigonometry
  Trigonometric Function9 : Trigonometry  Operator=cos
  abc : Outport
  wires:
  Constant8/1 -> Sum11/1
  Product7/1 -> Sum7/2
  Gain1/1 -> Mux1/2
  Product9/1 -> Sum8/2
  Sum7/1 -> Gain3/1
  Demux4/2 -> Product11/1  "q"
  Product10/1 -> Sum8/1
  Product11/1 -> Sum12/1
  Sum13/1 -> Trigonometric Function12/1
  Demux2/3 -> Trigonometric Function7/1, Trigonometric Function8/1
  Product12/1 -> Sum12/2
  Constant6/1 -> Sum10/1
  Product8/1 -> Sum7/1
  Mux1/1 -> abc/1
  Demux3/3 -> Sum9/2, Sum10/2
  Demux3/2 -> Product10/1  "q"
  Demux2/2 -> Product8/1  "q"
  dq/1 -> Mux/1
  Trigonometric Function7/1 -> Product7/2
  Constant5/1 -> Sum9/1
  Trigonometric Function12/1 -> Product12/2
  Trigonometric Function10/1 -> Product10/2
  Demux4/1 -> Product12/1  "d"
  Gain2/1 -> Mux1/3
  Demux4/3 -> Sum11/2, Sum13/2
  Demux2/1 -> Product7/1  "d"
  Sum10/1 -> Trigonometric Function10/1
  Gain3/1 -> Mux1/1
  Mux/1 -> Demux3/1, Demux2/1, Demux4/1
  Sum12/1 -> Gain2/1
  theta_d/1 -> Mux/2
  Sum11/1 -> Trigonometric Function11/1
  Trigonometric Function9/1 -> Product9/2
  Sum8/1 -> Gain1/1
  Sum9/1 -> Trigonometric Function9/1
  Demux3/1 -> Product9/1  "d"
  Trigonometric Function8/1 -> Product8/2
  Trigonometric Function11/1 -> Product11/2
  Constant7/1 -> Sum13/1

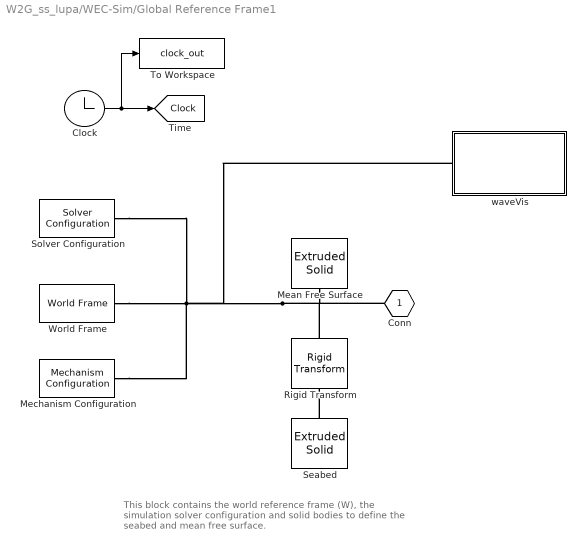
== system W2G_ss_lupa/WEC-Sim/Global Reference Frame1 ==
  note: This block contains the world reference frame (W), the simulation solver configuration and
      | solid bodies to define the seabed and mean free surface.
  Clock : Clock
  Mean Free Surface : sm_lib/Body Elements/Extruded Solid  GraphicAmbientColor=[0.15 0.15 0.15 1.0]  BasedOnType=Density  CenterOfMass=[0 0 0]  CenterOfMassUnits=m  GraphicDiffuseColor=[0.0 0.6 0.8]  ExportConvexHullGeometry=off  ExtrusionCrossSection=[simu.domainSize simu.domainSize; -simu.domainSize simu.domainSize; -simu.domainSize -simu.domainSize; simu.domainSize -simu.domainSize]  ExtrusionCrossSectionUnits=m  Density=1000  DensityUnits=kg/(m^3)  DoExposeReferenceFrame=on  GraphicEmissiveColor=[0.0 0.0 0.0 1.0]  ExportEntireGeometry=off  ExtrusionLength=simu.domainSize/200  ExtrusionLengthUnits=m  ExtrusionType=General  SerializedFrames=<Frames/>  MarkerShape=Sphere  MarkerSize=10  GraphicType=FromGeometry  InertiaType=Custom  Mass=10^20  MassUnits=kg  MomentsOfInertia=[10^20 10^20 10^20]  MomentsOfInertiaUnits=kg*m^2  PolygonNumSides=3  GraphicOpacity=0.3  PolygonOuterRadius=1  PolygonOuterRadiusUnits=m  ProductsOfInertia=[0 0 0]  ProductsOfInertiaUnits=kg*m^2  GraphicShininess=75  GraphicSpecularColor=[0.5 0.5 0.5 1.0]  GraphicVisPropType=SimpleVisualProperties
  Mechanism Configuration : sm_lib/Utilities/Mechanism Configuration  UniformGravity=Constant  GravityVector=[0 0 0]  GravityUnits=m/s^2  LinearizationDelta=0.001  JointModeTransitionNonlinearIterations=2
  Rigid Transform : sm_lib/Frames and Transforms/Rigid Transform  TranslationMethod=Cartesian  TranslationStandardOffset=0  TranslationLengthUnit=m  TranslationStandardAxis=+Z  TranslationCartesianOffset=[0 0 -waves.waterDepth]  TranslationROffset=0  TranslationROffsetUnits=m  TranslationZOffset=0  TranslationZOffsetUnits=m  TranslationThetaOffset=0  TranslationThetaOffsetUnits=deg  RotationMethod=None  RotationAngleUnits=deg  RotationStandardAxis=+Z  RotationAngle=0  RotationArbitraryAxis=[0 0 1]  FollAlignAxisA=+X  BaseAlignAxisA=+Y  FollAlignAxisB=+Y  BaseAlignAxisB=+Z  RotationSequenceAxes=FollowerAxes  RotationSequence=XYX  RotationSequenceAngles=[0 0 0]  RotationSequenceAnglesUnits=deg  RotationMatrix=[1 0 0; 0 1 0; 0 0 1]
  Seabed : sm_lib/Body Elements/Extruded Solid  GraphicAmbientColor=[0.15 0.15 0.15 1.0]  BasedOnType=Density  CenterOfMass=[0 0 0]  CenterOfMassUnits=m  GraphicDiffuseColor=[0.4 0.4 0.0]  ExportConvexHullGeometry=off  ExtrusionCrossSection=[simu.domainSize simu.domainSize; -simu.domainSize simu.domainSize; -simu.domainSize -simu.domainSize; simu.domainSize -simu.domainSize]  ExtrusionCrossSectionUnits=m  Density=1000  DensityUnits=kg/(m^3)  DoExposeReferenceFrame=on  GraphicEmissiveColor=[0.0 0.0 0.0 1.0]  ExportEntireGeometry=off  ExtrusionLength=simu.domainSize/100  ExtrusionLengthUnits=m  ExtrusionType=General  SerializedFrames=<Frames/>  MarkerShape=Sphere  MarkerSize=10  GraphicType=FromGeometry  InertiaType=Custom  Mass=10^20  MassUnits=kg  MomentsOfInertia=[10^20 10^20 10^20]  MomentsOfInertiaUnits=kg*m^2  PolygonNumSides=3  GraphicOpacity=1  PolygonOuterRadius=1  PolygonOuterRadiusUnits=m  ProductsOfInertia=[0 0 0]  ProductsOfInertiaUnits=kg*m^2  GraphicShininess=75  GraphicSpecularColor=[0.5 0.5 0.5 1.0]  GraphicVisPropType=SimpleVisualProperties
  Solver Configuration : nesl_utility/Solver Configuration  PhysicalDomain=network_engine_domain  SubClassName=solver  LeftPortType=input  RightPortType=generic  Tones=[]  Harmonics=[]  SimulateNoise=off  Profile=off  UseLocalSampling=off  EnableSwitchedLinearOptims=on  FrequencyDomain=off  UseCCode=off  RelTol=0.001  AbsTol=1e-06  MinStep=1e-09  ToWorkspace=off  RevertToSquareIcSolve=off  NumHomotopyIterations=100  PhasorMode=off  PhasorModeNumHarmonics=1  DoDC=on  ResidualTolerance=1e-9  UseLocalSolver=off  LocalSolverChoice=NE_BACKWARD_EULER_ADVANCER  LocalSolverSampleTime=.001  DoFixedCost=off  MaxNonlinIter=3  MaxModeIter=2  ComputeImpulses=off  ImpulseIterations=2  LinearAlgebra=Sparse  EquationFormulation=NE_TIME_EF  DelaysMemoryBudget=1024  AutomaticFiltering=on  FilteringTimeConstant=0.001  PartitionStorageMethod=AS_NEEDED  PartitionMemoryBudget=1024  PartitionMethod=FAST
      settings: SourceProductBaseCode=PW,SS
  To Workspace : ToWorkspace  VariableName=clock_out  SaveFormat=Structure With Time  SampleTime=-1
  World Frame : sm_lib/Frames and Transforms/World Frame
  waveVis : Subsystem  Variant=on  VariantControl=Choice  AllowZeroVariantControls=on  PropagateVariantConditions=on  mask{visualizationON=0}
      mask prompts: visualizationON "Visualization Option"
      mask init:
      | % sv_visulizationON  =Simulink.Variant('visualizationON');
      | % sv_visulizationOFF =Simulink.Variant('visualizationOFF');
      | 
      |     h = [gcb '/waveVisOff'];
      |     visualizationON = 'sv_visualizationOFF';
      |     set_param(h,'VariantControl',visualizationON);
      |     
      |     h = [gcb '/waveVisOn'];
      |     visualizationON = 'sv_visualizationON';
      |     set_param(h,'VariantControl',visualizationON);
      mask TypeOptions visualizationON: 0  | 1
  Conn : PMIOPort  Side=Right
  tag scope: Clock=global
  wires:
  Clock/1 -> [Clock], To Workspace/1
  connections:
  Seabed/RConn1 -- Rigid Transform/RConn1
  Solver Configuration/RConn1 -- Rigid Transform/LConn1 -- Mean Free Surface/RConn1 -- Conn/RConn1 -- waveVis/LConn1 -- Mechanism Configuration/RConn1 -- World Frame/RConn1

== system W2G_ss_lupa/WEC-Sim/Global Reference Frame1/waveVis ==
  waveVisOff : Subsystem  VariantControl=sv_visualizationOFF
  waveVisOn : Subsystem  VariantControl=sv_visualizationON
  Global Origin : PMIOPort  Side=Left

== system W2G_ss_lupa/WEC-Sim/Global Reference Frame1/waveVis/waveVisOff ==
  Global Origin : PMIOPort  Side=Left

== system W2G_ss_lupa/WEC-Sim/Global Reference Frame1/waveVis/waveVisOn ==
  water elevation : Subsystem  mask{waves=waves, wgloc=0, wgT=0}
      mask prompts: waves "Waves Object"; wgloc "Waves Gauge Location [X,Y]"; wgT "Waves Gauge Time History"
      mask init:
      | cb = gcb;
      | 
      | set_param([cb '/marker1'],...
      |            'position',[0,100,180,140]);
      | set_param([cb '/marker1'],...
      |            'wgloc',[sprintf('waves.marker.location(%d,:)',1)]); 
      | set_param([cb '/marker1'],...
      |            'wgT',[sprintf('[waves.waveAmpTimeViz(:,1), waves.waveAmpTimeViz(:,%d)]',2)]);
      | 
      | nGauges = size(waves.marker.location,1);
      | for iWG = 2:nGauges
      |     try 
      |         find_system([cb,'/marker',num2str(iWG)],'Type','Block');
      |     catch
      |         add_block([cb,'/marker1'],[cb,'/marker',num2str(iWG)],'MakeNameUnique','off',...
      |                    'Position',[0,100*iWG,180,40+100*iWG],'BackgroundColor','white');
      |         set_param([cb,'/marker',num2str(iWG)],'wgT',[sprintf('[waves.waveAmpTimeViz(:,1),waves.waveAmpTimeViz(:,%d)]',iWG+1)]);
      |         set_param([cb,'/marker',num2str(iWG)],'wgloc',[sprintf('waves.marker.location(%d,:)',iWG)]);
      |         add_line(cb,...
      |             ['marker',num2str(iWG),'/LConn1'],...
      |             ['Global Origin/RConn1'],...
      |             'autorouting','on');
      |     end
      | end
  Global Origin : PMIOPort  Side=Left
  connections:
  water elevation/LConn1 -- Global Origin/RConn1

== system W2G_ss_lupa/WEC-Sim/Global Reference Frame1/waveVis/waveVisOn/water elevation ==
  marker1 : Subsystem  mask{wgloc=waves.marker.location(1,:), wgT=[waves.waveAmpTimeViz(:,1), waves.waveAmpTimeViz(:,2)]}
      mask prompts: wgloc "Wave Gauge Location [X,Y]"; wgT "Wave Gauge Time History"
  Global Origin : PMIOPort  Side=Left
  connections:
  marker1/LConn1 -- Global Origin/RConn1

== system W2G_ss_lupa/WEC-Sim/Global Reference Frame1/waveVis/waveVisOn/water elevation/marker1 ==
  From Workspace : FromWorkspace  VariableName=wgT
  Rigid Transform : sm_lib/Frames and Transforms/Rigid Transform  TranslationMethod=Cartesian  TranslationStandardOffset=0  TranslationLengthUnit=m  TranslationStandardAxis=+Z  TranslationCartesianOffset=[wgloc 0]  TranslationROffset=0  TranslationROffsetUnits=m  TranslationZOffset=0  TranslationZOffsetUnits=m  TranslationThetaOffset=0  TranslationThetaOffsetUnits=deg  RotationMethod=None  RotationAngleUnits=deg  RotationStandardAxis=+Z  RotationAngle=0.0  RotationArbitraryAxis=[0 0 1]  FollAlignAxisA=+X  BaseAlignAxisA=+Y  FollAlignAxisB=+Y  BaseAlignAxisB=+Z  RotationSequenceAxes=FollowerAxes  RotationSequence=XYX  RotationSequenceAngles=[0 0 0]  RotationSequenceAnglesUnits=deg  RotationMatrix=[1 0 0; 0 1 0; 0 0 1]
  Visualization Block : Subsystem  mask{markStyle=waves.marker.style, markSize=waves.marker.size}
      mask prompts: markStyle "Waves Marker Style"; markSize "Waves Marker Size"
      mask init:
      | % Marker Shape %<MarkerShape>
      | % Marker Size %<MarkerSize>%<MarkerSizeUnits>
      | cb = gcb;
      | 
      | set_param([cb '/WaveElevation'],'MarkerSize','markSize')
      | 
      | if markStyle == 1
      |     set_param([cb '/WaveElevation'],'MarkerShape','Sphere')
      | elseif markStyle == 2
      |     set_param([cb '/WaveElevation'],'MarkerShape','Cube')
      | elseif markStyle == 3
      |     set_param([cb '/WaveElevation'],'MarkerShape','Frame')
      | end
  Conn1 : PMIOPort  Side=Left
  wires:
  From Workspace/1 -> Visualization Block/1(Input)
  connections:
  Rigid Transform/LConn1 -- Conn1/RConn1
  Rigid Transform/RConn1 -- Visualization Block/LConn1

== system W2G_ss_lupa/WEC-Sim/Global Reference Frame1/waveVis/waveVisOn/water elevation/marker1/Visualization Block ==
  Input : Inport
  Derivative : Derivative
  Derivative1 : Derivative
  Simulink-PS Converter : nesl_utility/Simulink-PS Converter  PhysicalDomain=network_engine_domain  SubClassName=ps_input  LeftPortType=input  RightPortType=output  PseudoPeriodic=off  Frequencies=[]  NoiseDistribution=none  NoiseParameters=[]  Unit=1  AffineConversion=off  FilteringAndDerivatives=provide  SimscapeFilterOrder=1  InputFilterTimeConstant=0.001  UdotUserProvided=2
      settings: SourceProductBaseCode=PW,SS
  WaveElevation : sm_lib/Body Elements/Graphic  GraphicType=Marker  MarkerShape=Sphere  MarkerSize=markSize  GraphicVisPropType=SimpleVisualProperties  GraphicDiffuseColor=[0.2 1.0 0.6]  GraphicSpecularColor=[0.5 0.5 0.5 1.0]  GraphicAmbientColor=[0.15 0.15 0.15 1.0]  GraphicEmissiveColor=[0.0 0.0 0.0 1.0]  GraphicShininess=75  GraphicOpacity=1.0
      settings: AttributesFormatString=|
      | Marker Shape: %<MarkerShape>
      | Marker Size:    %<MarkerSize>%<MarkerSizeUnits>
  eta : sm_lib/Joints/Prismatic Joint  JointMode=Normal  SenseConstraintForce=off  SenseConstraintForceX=off  SenseConstraintForceY=off  SenseConstraintForceZ=off  SenseConstraintTorque=off  SenseConstraintTorqueX=off  SenseConstraintTorqueY=off  SenseConstraintTorqueZ=off  SenseTotalForce=off  SenseTotalForceX=off  SenseTotalForceY=off  SenseTotalForceZ=off  SenseTotalTorque=off  SenseTotalTorqueX=off  SenseTotalTorqueY=off  SenseTotalTorqueZ=off  CompositeWrenchDir=FollowerOnBase  CompositeWrenchFrame=BaseFrame  EquilibriumPosition=0  EquilibriumPositionUnits=m  SpringStiffness=0  SpringStiffnessUnits=N/m  DampingCoefficient=0  DampingCoefficientUnits=N/(m/s)  TorqueActuationMode=ComputedTorque  MotionActuationMode=InputMotion  SensePosition=off  SenseVelocity=off  SenseAcceleration=off  SenseTorqueForce=off  SenseLowerLimitTorqueForce=off  SenseUpperLimitTorqueForce=off  LowerLimitSpecify=off  LowerLimitBound=-1  LowerLimitBoundUnits=m  LowerLimitStiffness=1e6  LowerLimitStiffnessUnits=N/m  LowerLimitDamping=1e3  LowerLimitDampingUnits=N/(m/s)  LowerLimitTransitionRegionWidth=1e-4  LowerLimitTransitionRegionWidthUnits=m  UpperLimitSpecify=off  UpperLimitBound=1  UpperLimitBoundUnits=m  UpperLimitStiffness=1e6  UpperLimitStiffnessUnits=N/m  UpperLimitDamping=1e3  UpperLimitDampingUnits=N/(m/s)  UpperLimitTransitionRegionWidth=1e-4  UpperLimitTransitionRegionWidthUnits=m  PositionTargetSpecify=off  PositionTargetPriority=High  PositionTargetValue=0  PositionTargetValueUnits=m  VelocityTargetSpecify=off  VelocityTargetPriority=High  VelocityTargetValue=0  VelocityTargetValueUnits=m/s
  Conn1 : PMIOPort  Side=Left
  wires:
  Derivative1/1 -> Simulink-PS Converter/3
  Derivative/1 -> Simulink-PS Converter/2, Derivative1/1
  Input/1 -> Simulink-PS Converter/1, Derivative/1
  connections:
  eta/LConn1 -- Conn1/RConn1
  WaveElevation/RConn1 -- eta/RConn1
  Simulink-PS Converter/RConn1 -- eta/LConn2

== matlab function W2G_ss_lupa/Linear Generator & AC//DC Converter (S.S. model)/S.S. Motor and Drive Model Q=0/convert nan to zero ==
  data: u input; y output
function y = fcn(u)
if isnan(u)
    y=0;
else
    y = u;
end
end

== matlab function W2G_ss_lupa/Linear Generator & AC//DC Converter (S.S. model)/S.S. Motor and Drive Model Q=0/convert nan to 0 ==
  data: u input; y output
function y = fcn(u)
if isnan(u)
    y=0;
else
    y = u;
end
end
